simulink library "cdmalibv1p1"  (Simulink 5.0)
undefined symbols (not defined in the file or in its folder): M, N
libraries: cdmalibv1p1 x28, dspsigops x13, dspbuff3 x8, simulink3 x4, commutil2 x3, commsequence2 x1
settings Model: CovMetricSettings=d  Creator=pc  LastModifiedBy=jli

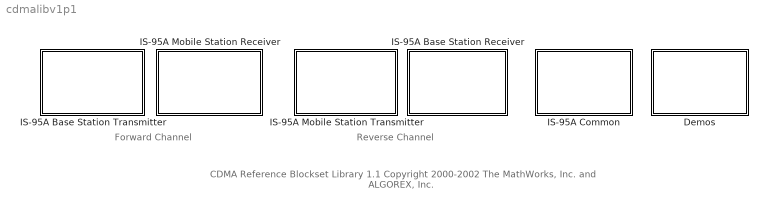
== system cdmalibv1p1 ==
  note: CDMA Reference Blockset Library 1.1
      | Copyright 2000-2002 The MathWorks, Inc. and ALGOREX, Inc.
  note: Forward Channel
  note: Reverse Channel
  Demos : Subsystem
      settings: OpenFcn=demo blocksets CDMA
      mask Type: DSP Demos
      mask Display: disp('Demos')
  IS-95A Base Station Receiver : Subsystem
      mask Display: disp('IS-95A \nBase Station\nReceiver')
  IS-95A Base Station Transmitter : Subsystem
      mask Display: disp('IS-95A \nBase Station\nTransmitter')
  IS-95A Common : Subsystem
      mask Display: disp('IS-95A \nCommon')
  IS-95A Mobile Station Receiver : Subsystem
      mask Display: disp('IS-95A \nMobile Station\nReceiver')
  IS-95A Mobile Station Transmitter : Subsystem
      mask Display: disp('IS-95A \nMobile Station\nTransmitter')

== system cdmalibv1p1/Demos ==

== system cdmalibv1p1/IS-95A Base Station Receiver ==
  IS-95A Rev Ch Viterbi Decoder : S-Function  FunctionName=sis95rcdec  Parameters=rateSet chType traceBackLenRatio decodeLenRatio  mask(IS-95A Rev Ch Viterbi Decoder){rateSet=Rate Set I, chType=Traffic, traceBackLenRatio=1, decodeLenRatio=1}
      mask prompts: rateSet "Rate set:"; chType "Channel type:"; traceBackLenRatio "Ratio of trace-back length to frame length:"; decodeLenRatio "Ratio of decoding length to frame length:"
      mask help: Perform optimum decoding for a convolutionally encoded reverse Access or Traffic channel frame.
      mask Help: web(cdmaweb);
      mask StyleString: popup(Rate Set I|Rate Set II),popup(Access|Traffic),edit,edit
      mask Display:
      | port_label('input', 1, 'Rate');
      | port_label('input', 2, 'Frame In');
      | port_label('output', 2, 'Metric');
      | port_label('output', 1, 'Frame Out');
  IS-95A Rev Ch Walsh Correlator : S-Function  FunctionName=sis95rcwalshcor  Parameters=wlshOrd numSymb  mask(IS-95A Rev Ch Walsh Correlator){wlshOrd=6, numSymb=1}
      mask prompts: wlshOrd "Walsh order:"; numSymb "Number of input symbols:"
      mask help:
      | Correlate the input sequence with a bank of Walsh sequences for the reverse Access or Traffic channel frame. The length of the input vector is
      | (Number of input symbols) * (2^Walsh order).
      mask Help: web(cdmaweb);
      mask Display: disp('IS-95A Rev Ch \nWalsh Correlator');
  IS-95A Rev Ch Walsh Demodulator : S-Function  FunctionName=sis95rcwalshdemod  Parameters=wlshOrd numSymb  mask(IS-95A Rev Ch Walsh Demodulator){wlshOrd=6, numSymb=1}
      mask prompts: wlshOrd "Walsh order:"; numSymb "Number of input symbols:"
      mask help: Perform Walsh demodulation of the received signal. The length of the input vector is (Number of input symbols) * (2^Walsh order).
      mask Help: web(cdmaweb);
      mask Display:
      | port_label('output', 1, 'Hard Dec');
      | port_label('output', 2, 'Soft Dec');
  IS-95A Rev Ch  Rake Finger : Subsystem  TreatAsAtomicUnit=on  mask(IS-95A Rev Ch Rake Finger){wlshOrd=6, outSize=1, buffSize=3, ovrSmp=8}
      mask prompts: wlshOrd "Walsh order:"; outSize "Output size (in number of walsh functions):"; buffSize "Tracking buffer size (in number of symbols):"; ovrSmp "Oversampling rate:"
      mask help: Despread the received signal with the short PN and long codes and then correlate the despread signal with all of the Walsh code sequences.
      mask Help: web(cdmaweb);
  IS-95A Rev Ch Detector : Subsystem  mask(IS-95A Rev Ch Detector){chType=Traffic, wlshOrd=6, lngcd_mask=2^41, overSamplRate=8, sampTime=1/(50*384)}
      mask prompts: chType "Channel type:"; wlshOrd "Walsh order:"; lngcd_mask "Long code mask:"; overSamplRate "Oversampling rate:"; sampTime "Sample time:"
      mask help: Perform noncoherent detection of the reverse Access or Traffic channel frame.
      mask init:
      | is95noncohdetector;
      mask Help: web(cdmaweb);
      mask StyleString: popup(Access|Traffic),edit,edit,edit,edit
  IS-95A Rev Ch Short Code Despreader : S-Function  FunctionName=sis95rcdespread  Parameters=numSymb buffSize integLen ovrSmp  mask(IS-95A Rev Ch Short Code Despreader){numSymb=1, integLen=64, buffSize=3, ovrSmp=8}
      mask prompts: numSymb "Input frame size (in number of symbols):"; integLen "Walsh size:"; buffSize "Tracking buffer size (in number of symbols):"; ovrSmp "Oversampling rate:"
      mask help: Perform despreading of the input I and Q frames with the I and Q short PN codes.
      mask Help: web(cdmaweb);
      mask Display:
      | port_label('input', 1, 'Rx I');
      | port_label('input', 2, 'Rx Q');
      | port_label('input', 3, 'PN I');
      | port_label('input', 4, 'PN Q');
      | port_label('input', 5, 'Path Delay');
      | port_label('output', 1, 'Data I');
      | port_label('output', 2, 'Data Q');

== system cdmalibv1p1/IS-95A Base Station Transmitter ==
  IS-95A Fwd Ch Convolutional Encoder : S-Function  FunctionName=sis95enc  Parameters=ch_type rate_set enc_state  mask(IS-95A Fwd Ch Convolutional Encoder){rate_set=Rate Set I, ch_type=Traffic, enc_state=[]}
      mask prompts: rate_set "Rate set:"; ch_type "Channel type:"; enc_state "Initial encoder state:"
      mask help: Convolutionally encode the bits of the forward Sync, Paging or Traffic channel frame.
      mask Help: web(cdmaweb);
      mask StyleString: popup(Rate Set I|Rate Set II),popup(Sync|Paging|Traffic),edit
      mask Display:
      | port_label('input', 1, 'Rate');
      | port_label('input', 2, 'Frame In');
  IS-95A Fwd Ch Interleaver/Deinterleaver : S-Function  FunctionName=sis95int  Parameters=ch_type intlv_tbl int_option  mask(IS-95A Fwd Ch Interleaver/Deinterleaver){ch_type=Traffic, int_select=Interleaver}
      mask prompts: ch_type "Channel type:"; int_select "Function:"
      mask help: Interleave or deinterleave the symbols of the forward Sync, Paging or Traffic Channel frame.
      mask init:
      | is95fwdchinterleaver;
      mask Help: web(cdmaweb);
      mask StyleString: popup(Sync|Paging|Traffic),popup(Interleaver|Deinterleaver)
      mask Display: disp('IS-95A Fwd Ch \nInterleaver/\nDeinterleaver');
  IS-95A Fwd Ch Repeater/Derepeater : S-Function  FunctionName=sis95rep  Parameters=ch_type rate_set rep_option  mask(IS-95A Fwd Ch Repeater/Derepeater){rate_set=Rate Set I, ch_type=Traffic, rep_select=Derepeater}
      mask prompts: rate_set "Rate set:"; ch_type "Channel type:"; rep_select "Function:"
      mask help: Repeat and puncture if necessary or derepeat the symbols of a convolutionally encoded frame for the forward Sync, Paging or Traffic channel.
      mask init:
      | is95fwdchrepeater;
      mask Help: web(cdmaweb);
      mask StyleString: popup(Rate Set I|Rate Set II),popup(Sync|Paging|Traffic),popup(Repeater|Derepeater)
      mask Display:
      | port_label('input', 1, 'Rate');
      | port_label('input', 2, 'Frame In');
  IS-95A Fwd Ch Scrambler : S-Function  FunctionName=sis95scramble  Parameters="chType  rate_set"  mask(IS-95A Fwd Ch Scrambler){rate_set=Rate Set I, chType=Traffic}
      mask prompts: rate_set "Rate set:"; chType "Channel type:"
      mask help: Scramble the symbols of the forward Paging or Traffic channel frame by the decimated long code and insert power control bits into the Traffic channel frame.
      mask Help: web(cdmaweb);
      mask StyleString: popup(Rate Set I|Rate Set II),popup(Sync|Paging|Traffic)
      mask Display:
      | port_label('input', 1, 'Rate');
      | port_label('input', 2, 'Data In');
      | port_label('input', 3, 'Long Code');
      | port_label('input', 4, 'Power Bits');
  IS-95A Fwd Ch Base Station Transmitter Interface : Subsystem  mask(IS-95A Fwd Ch Base Station Transmitter Interface){paging_rate=Full, wlshOrd=6, wlsh_indices=[0 32 2 38 23], sampTime=1/(50*384)}
      mask prompts: paging_rate "Paging channel rate:"; wlshOrd "Walsh order:"; wlsh_indices "Pilot, sync, paging, traffic and OCNS Walsh indices:"; sampTime "Sample time:"
      mask help: Combine Pilot, Sync, Paging, Traffic and Orthogonal Channel Noise Simulator (OCNS) symbols using different Walsh Code sequences.
      mask Help: web(cdmaweb);
      mask StyleString: popup(Full|Half),edit,edit,edit

== system cdmalibv1p1/IS-95A Common ==
  IS-95A CRC Generator : S-Function  FunctionName=sis95crcgen  Parameters=ch_type rate_set 1  mask(IS-95A CRC Generator){rate_set=Rate Set I, ch_type=Traffic}
      mask prompts: rate_set "Rate set:"; ch_type "Channel type:"
      mask help: Generate Cyclic Redundancy Check (CRC) bits and add them along with the tail bits to the forward or reverse Traffic channel frame.
      mask Help: web(cdmaweb);
      mask StyleString: popup(Rate Set I|Rate Set II),popup(Sync|Paging|Access|Traffic)
      mask Display:
      | port_label('input', 1, 'Rate');
      | port_label('input', 2, 'Frame In');
  IS-95A Frame Quality  Detector : Subsystem  mask(IS-95A Frame Quality Detector){rateSet=Rate Set I, chType=Traffic, rate2_metric=0.9*1.5, rate3_metric=0.85*1.5}
      mask prompts: rateSet "Rate set:"; chType "Channel type:"; rate2_metric "Metric threshold for quarter rate:"; rate3_metric "Metric threshold for eighth rate:"
      mask help: Determine the quality of a received frame of data and output the decoded data and a frame quality indicator.
      mask init:
      | is95framequalitydet;
      mask Help: web(cdmaweb);
      mask StyleString: popup(Rate Set I|Rate Set II),popup(Sync|Paging|Access|Traffic),edit,edit
  IS-95A Long Code Generator : S-Function  FunctionName=sis95lcgen2  Parameters="tx_sample_time tx_lc_init_state tx_lc_init_mask tx_lc_dec_ratio  num_symb"  mask(IS-95A Long Code Generator){num_symb=4, tx_lc_dec_ratio=1, tx_lc_init_mask=2^41, tx_lc_init_state=2^41, tx_sample_time=1/(50*384)}
      mask prompts: num_symb "Output frame size:"; tx_lc_dec_ratio "Decimation ratio:"; tx_lc_init_mask "Long code mask:"; tx_lc_init_state "Initial state:"; tx_sample_time "Sample time:"
      mask help: Generate the long code sequence used for reverse channel spreading and scrambling and forward channel scrambling.
      mask init:
      | is95longcodegenerator;
      mask Help: web(cdmaweb);
      mask Display: disp('IS-95A Long \nCode Generator');
  IS-95A Short Code Generator : S-Function  FunctionName=sis95scgen2  Parameters=numOut sampTime  mask(IS-95A Short Code Generator){numOut=64, sampTime=1/(50*384)}
      mask prompts: numOut "Output frame size:"; sampTime "Sample time:"
      mask help: Generate the I and Q short PN code sequences that are used to perform quadrature spreading of the forward or reverse channel frame. The input is a mask that determines the output of the I and Q short PN codes.
      mask Help: web(cdmaweb);
      mask Display:
      | port_label('output', 1, 'PN I');
      | port_label('output', 2, 'PN Q');
  IS-95A Syndrome Detector : S-Function  FunctionName=sis95crcgen  Parameters=chType rate_set 0  mask(IS-95A Syndrome Detector){rate_set=Rate Set I, chType=Traffic}
      mask prompts: rate_set "Rate set:"; chType "Channel type:"
      mask help: Check the CRC bits to determine the frame quality and output the decoded data and frame quality decision for all forward or reverse channels.
      mask Help: web(cdmaweb);
      mask StyleString: popup(Rate Set I|Rate Set II),popup(Sync|Paging|Access|Traffic)
      mask Display:
      | port_label('input', 1, 'Rate');
      | port_label('input', 2, 'Frame In');
      | port_label('output', 1, 'Frame Out');
      | port_label('output', 2, 'Frame Error');
  IS-95A Walsh Code Generator : S-Function  FunctionName=sis95wcgen2  Parameters=wlshOrd wlshIndices st  mask(IS-95A Walsh Code Generator){wlshOrd=6, wlshIndices=[0 32 2 38 23], st=1/(50*384)}
      mask prompts: wlshOrd "Walsh order:"; wlshIndices "Walsh indices:"; st "Sample time:"
      mask help: Generate the Walsh code sequences corresponding to the specified Walsh order and indices.
      mask Help: web(cdmaweb);
      mask Display: disp('IS-95A Walsh \nCode Generator');

== system cdmalibv1p1/IS-95A Mobile Station Receiver ==
  IS-95A Fwd Ch Descrambler : Subsystem  mask(IS-95A Fwd Ch Descrambler){rateSet=Rate Set I, rake_buff_size=3}
      mask prompts: rateSet "Rate set:"; rake_buff_size "Tracking buffer size:"
      mask help: Perform power bit extraction and descrambling for each rake finger and combine the signals from all the fingers.
      mask init:
      | is95fwdchdescramble;
      mask Help: web(cdmaweb);
      mask StyleString: popup(Rate Set I|Rate Set II),edit
  IS-95A Fwd Ch Power Bit Extractor : Subsystem  TreatAsAtomicUnit=on  mask(IS-95A Fwd Ch Power Bit Extractor){rateSet=Rate Set I, num_symb=1, init_loc=0}
      mask prompts: rateSet "Rate set:"; num_symb "Input frame size:"; init_loc "Initial power bit location:"
      mask help: Extract power control bits from the forward Traffic channel frame.
      mask init:
      | is95fwdchpwrbitext;
      mask Help: web(cdmaweb);
      mask StyleString: popup(Rate Set I|Rate Set II),edit,edit
  IS-95A Fwd Ch Rake Demodulator : S-Function  FunctionName=sis95rakedemod  Parameters=num_symb 4  mask(IS-95A Fwd Ch Rake Demodulator){num_symb=1}
      mask prompts: num_symb "Input frame size per finger:"
      mask help: Demodulate the data obtained from the four rake receiver fingers utilizing the pilot signal for each finger.
      mask Help: web(cdmaweb);
      mask Display:
      | port_label('input', 1, 'Pilot I');
      | port_label('input', 2, 'Pilot Q');
      | port_label('input', 3, 'Data I');
      | port_label('input', 4, 'Data Q');
      | port_label('output', 1, 'Finger 1');
      | port_label('output', 2, 'Finger 2');
      | port_label('output', 3, 'Finger 3');
      | port_label('output', 4, 'Finger 4');
  IS-95A Fwd Ch Viterbi Decoder : S-Function  FunctionName=sis95dec  Parameters=rateSet chType traceBackLenRatio decodeLenRatio  mask(IS-95A Fwd Ch Viterbi Decoder){rateSet=Rate Set I, chType=Traffic, traceBackLenRatio=1, decodeLenRatio=1}
      mask prompts: rateSet "Rate set:"; chType "Channel type:"; traceBackLenRatio "Ratio of trace-back length to frame length:"; decodeLenRatio "Ratio of decoding length to frame length:"
      mask help: Perform optimum decoding for a convolutionally encoded forward Sync, Paging or Traffic channel frame.
      mask Help: web(cdmaweb);
      mask StyleString: popup(Rate Set I|Rate Set II),popup(Sync|Paging|Traffic),edit,edit
      mask Display:
      | port_label('input', 1, 'Rate');
      | port_label('input', 2, 'Frame In');
      | port_label('output', 2, 'Metric');
      | port_label('output', 1, 'Frame Out');
  IS-95A Fwd Ch  Rake Finger : Subsystem  TreatAsAtomicUnit=on  mask(IS-95A Fwd Ch Rake Finger){wlshOrd=6, numSymb=1, buffSize=3, ovrSmp=8}
      mask prompts: wlshOrd "Walsh order:"; numSymb "Input frame size (in number of symbols):"; buffSize "Tracking buffer size (in number of symbols):"; ovrSmp "Oversampling rate:"
      mask help: Correlate the input signal over each Walsh code interval with the short PN code and the Walsh code sequences supplied.
      mask init:
      | is95fwdchrakefinger;
      mask Help: web(cdmaweb);
  IS-95A Fwd Ch Detector : Subsystem  mask(IS-95A Fwd Ch Detector){rateSet=Rate Set I, numSymb=1, wlshOrd=6, rake_buff_size=3, rake_oversamp=8, sampTime=1/(50*384)}
      mask prompts: rateSet "Rate set:"; numSymb "Input frame size (in number of symbols):"; wlshOrd "Walsh order:"; rake_buff_size "Tracking buffer size (in number of symbols):"; rake_oversamp "Oversampling rate:"; sampTime "Sample time:"
      mask help: Perform despreading, demodulation and rake combining of the received signal.
      mask init:
      | is95cohdetector;
      mask Help: web(cdmaweb);
      mask StyleString: popup(Rate Set I|Rate Set II),edit,edit,edit,edit,edit

== system cdmalibv1p1/IS-95A Mobile Station Transmitter ==
  IS-95A Rev Ch Burst Randomizer : S-Function  FunctionName=sis95rcrandomizer  Parameters=chType initLCSt  mask(IS-95A Rev Ch Burst Randomizer){chType=Traffic, initLCSt=[]}
      mask prompts: chType "Channel type:"; initLCSt "Randomizer initial state:"
      mask help: Generate a pseudorandom masking pattern of 0's and 1's that can be used to mask redundant power groups.
      mask Help: web(cdmaweb);
      mask StyleString: popup(Access|Traffic),edit
      mask Display:
      | port_label('input', 1, 'Rate');
      | port_label('input', 2, 'Long Code');
  IS-95A Rev Ch Convolutional Encoder : S-Function  FunctionName=sis95rcenc  Parameters=ch_type rate_set enc_state  mask(IS-95A Rev Ch Convolutional Encoder){rate_set=Rate Set I, ch_type=Traffic, enc_state=[]}
      mask prompts: rate_set "Rate set:"; ch_type "Channel type:"; enc_state "Initial encoder state:"
      mask help: Convolutionally encode the bits of the reverse Access or Traffic channel frame.
      mask Help: web(cdmaweb);
      mask StyleString: popup(Rate Set I|Rate Set II),popup(Access|Traffic),edit
      mask Display:
      | port_label('input', 1, 'Rate');
      | port_label('input', 2, 'Frame In');
  IS-95A Rev Ch Interleaver/Deinterleaver : S-Function  FunctionName=sis95rcint  Parameters=ch_type rlinttable int_option  mask(IS-95A Rev Ch Interleaver/Deinterleaver){ch_type=Traffic, int_select=Interleaver}
      mask prompts: ch_type "Channel type:"; int_select "Function:"
      mask help: Interleave or deinterleave the symbols of the reverse Access or Traffic channel frame.
      mask init:
      | is95revchinterleaver;
      mask Help: web(cdmaweb);
      mask StyleString: popup(Access|Traffic),popup(Interleaver|Deinterleaver)
      mask Display:
      | port_label('input', 1, 'Rate');
      | port_label('input', 2, 'Frame In');
  IS-95A Rev Ch Repeater/Derepeater : S-Function  FunctionName=sis95rcrep  Parameters=ch_type rep_option  mask(IS-95A Rev Ch Repeater/Derepeater){ch_type=Traffic, rep_select=Derepeater}
      mask prompts: ch_type "Channel type:"; rep_select "Function:"
      mask help: Repeat or derepeat the symbols of the convolutionally encoded frame for the reverse Access or Traffic channel.
      mask init:
      | is95revchrepeater;
      mask Help: web(cdmaweb);
      mask StyleString: popup(Access|Traffic),popup(Repeater|Derepeater)
      mask Display:
      | port_label('input', 1, 'Rate');
      | port_label('input', 2, 'Frame In');
  IS-95A Rev Ch Walsh Modulator : S-Function  FunctionName=sis95walshmod  Parameters=walshOrder numSymb  mask(IS-95A Rev Ch Walsh Modulator){walshOrder=6, numSymb=6}
      mask prompts: walshOrder "Walsh order:"; numSymb "Input vector length:"
      mask help:
      | Modulate the input data symbols with the Walsh code sequences.
      | The length of the input vector must be an integer multiple of the Walsh order.
      mask Help: web(cdmaweb);
      mask Display: disp('IS-95A Rev Ch \nWalsh Modulator');
  IS-95A Rev Ch Walsh Modulation and Spreading : Subsystem  mask(IS-95A Rev Ch Walsh Modulation and Spreading){chType=Traffic, lngCdMask=1, wlshOrd=6, sampTime=1/(50*384)}
      mask prompts: chType "Channel type:"; lngCdMask "Long code mask:"; wlshOrd "Walsh order:"; sampTime "Sample time:"
      mask help: Perform Walsh code modulation, spreading with the long code, and power group randomization on a reverse Access or Traffic channel frame.
      mask init:
      | is95revchmodspread;
      mask Help: web(cdmaweb);
      mask StyleString: popup(Access|Traffic),edit,edit,edit

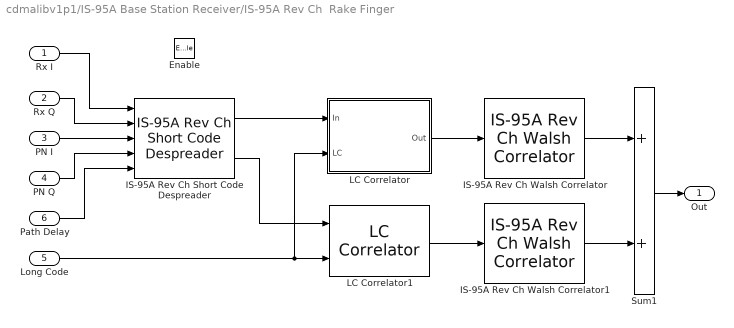
== system cdmalibv1p1/IS-95A Base Station Receiver/IS-95A Rev Ch  Rake Finger ==
  Rx I : Inport
  Rx Q : Inport  Port=2
  PN I : Inport  Port=3
  PN Q : Inport  Port=4
  Long Code : Inport  Port=5
  Path Delay : Inport  Port=6
  Enable : EnablePort
  IS-95A Rev Ch Walsh Correlator : cdmalibv1p1/IS-95A Base Station Receiver/IS-95A Rev Ch Walsh Correlator  wlshOrd=wlshOrd  numSymb=outSize
  IS-95A Rev Ch Walsh Correlator1 : cdmalibv1p1/IS-95A Base Station Receiver/IS-95A Rev Ch Walsh Correlator  wlshOrd=wlshOrd  numSymb=outSize
  IS-95A Rev Ch Short Code Despreader : cdmalibv1p1/IS-95A Base Station Receiver/IS-95A Rev Ch Short Code Despreader  numSymb=outSize  integLen=2^wlshOrd  buffSize=buffSize  ovrSmp=ovrSmp
  LC Correlator : Subsystem
  LC Correlator1 : cdmalibv1p1/IS-95A Base Station Receiver/IS-95A Rev Ch  Rake Finger/LC Correlator
      settings: RTWFcnNameOpts=Auto  RTWFileNameOpts=Auto
  Sum1 : Sum  SaturateOnIntegerOverflow=on  InputSameDT=on
  Out : Outport  InitialOutput=0
  wires:
  Long Code/1 -> LC Correlator/2(LC), LC Correlator1/2
  IS-95A Rev Ch Short Code Despreader/1 -> LC Correlator/1(In)
  Path Delay/1 -> IS-95A Rev Ch Short Code Despreader/5
  PN Q/1 -> IS-95A Rev Ch Short Code Despreader/4
  PN I/1 -> IS-95A Rev Ch Short Code Despreader/3
  Rx Q/1 -> IS-95A Rev Ch Short Code Despreader/2
  Rx I/1 -> IS-95A Rev Ch Short Code Despreader/1
  IS-95A Rev Ch Short Code Despreader/2 -> LC Correlator1/1
  IS-95A Rev Ch Walsh Correlator/1 -> Sum1/1
  Sum1/1 -> Out/1
  IS-95A Rev Ch Walsh Correlator1/1 -> Sum1/2
  LC Correlator1/1 -> IS-95A Rev Ch Walsh Correlator1/1
  LC Correlator/1(Out) -> IS-95A Rev Ch Walsh Correlator/1

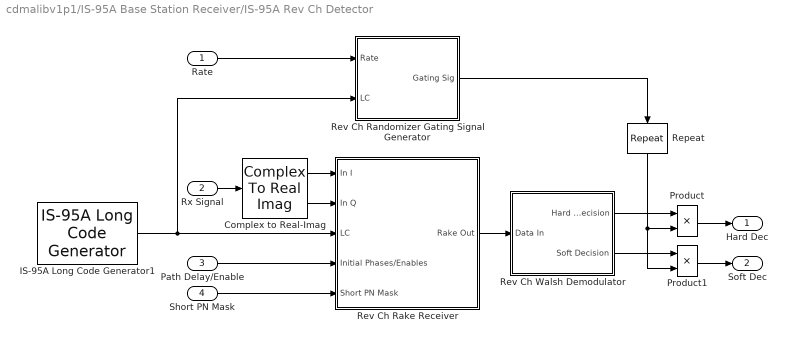
== system cdmalibv1p1/IS-95A Base Station Receiver/IS-95A Rev Ch Detector ==
  Rate : Inport
  Rx Signal : Inport  Port=2
  Path Delay/Enable : Inport  Port=3
  Short PN Mask : Inport  Port=4
  Complex to Real-Imag : ComplexToRealImag
  IS-95A Long Code Generator1 : cdmalibv1p1/IS-95A Common/IS-95A Long Code Generator  num_symb=N*(2^wlshOrd)*4  tx_lc_dec_ratio=1  tx_lc_init_mask=lngcd_mask  tx_lc_init_state=[]  tx_sample_time=N*4*sampTime
  Product : Product  SaturateOnIntegerOverflow=on  InputSameDT=on
  Product1 : Product  SaturateOnIntegerOverflow=on  InputSameDT=on
  Repeat : dspsigops/Repeat  Orientation=down  N=36  ic=0  mode=Maintain input frame rate
  Rev Ch Rake Receiver : Subsystem
  Rev Ch Randomizer Gating Signal Generator : Subsystem
  Rev Ch Walsh Demodulator : Subsystem  mask(IS95A NonCoh Walsh Demod){inSize=N, off=(M+1)*N, wlshOrder=wlshOrd}
      mask prompts: inSize "Input Size (in No of Walsh Functions)"; off "Input Delay (in No of Walsh Functions)"; wlshOrder "Walsh Order"
      mask help: Performs Walsh demodulation of the signal after combining the output of the rake fingers.
      mask Help: web(cdmaweb);
  Hard Dec : Outport  InitialOutput=0
  Soft Dec : Outport  Port=2  InitialOutput=0
  wires:
  IS-95A Long Code Generator1/1 -> Rev Ch Rake Receiver/3(LC), Rev Ch Randomizer Gating Signal Generator/2(LC)
  Complex to Real-Imag/1 -> Rev Ch Rake Receiver/1(In I)
  Rev Ch Randomizer Gating Signal Generator/1(Gating Sig) -> Repeat/1
  Complex to Real-Imag/2 -> Rev Ch Rake Receiver/2(In Q)
  Path Delay/Enable/1 -> Rev Ch Rake Receiver/4(Initial Phases/Enables)
  Rev Ch Rake Receiver/1(Rake Out) -> Rev Ch Walsh Demodulator/1(Data In)
  Short PN Mask/1 -> Rev Ch Rake Receiver/5(Short PN Mask)
  Rx Signal/1 -> Complex to Real-Imag/1
  Repeat/1 -> Product/2, Product1/2
  Rev Ch Walsh Demodulator/2(Soft Decision) -> Product1/1
  Rev Ch Walsh Demodulator/1(Hard Decision) -> Product/1
  Product/1 -> Hard Dec/1
  Product1/1 -> Soft Dec/1
  Rate/1 -> Rev Ch Randomizer Gating Signal Generator/1(Rate)

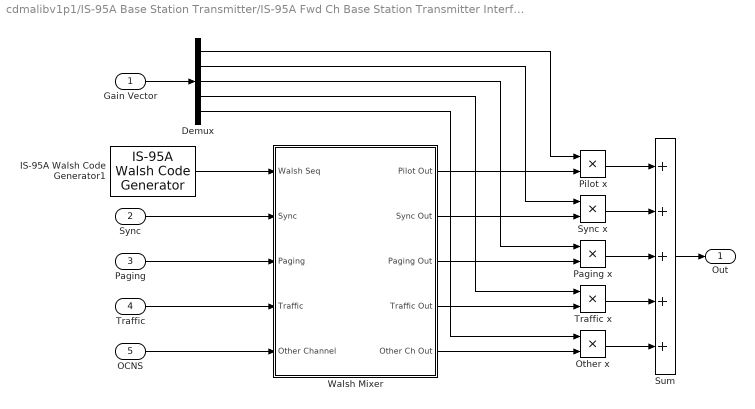
== system cdmalibv1p1/IS-95A Base Station Transmitter/IS-95A Fwd Ch Base Station Transmitter Interface ==
  Gain Vector : Inport
  Sync : Inport  Port=2
  Paging : Inport  Port=3
  Traffic : Inport  Port=4
  OCNS : Inport  Port=5
  Demux : Demux  Outputs=5
  IS-95A Walsh Code Generator1 : cdmalibv1p1/IS-95A Common/IS-95A Walsh Code Generator  wlshOrd=wlshOrd  wlshIndices=wlsh_indices  st=sampTime
  Other x : Product  Inputs=**  SaturateOnIntegerOverflow=on  InputSameDT=on
  Paging x : Product  Inputs=**  SaturateOnIntegerOverflow=on  InputSameDT=on
  Pilot x : Product  Inputs=**  SaturateOnIntegerOverflow=on  InputSameDT=on
  Sum : Sum  Inputs=+++++  SaturateOnIntegerOverflow=on  InputSameDT=on
  Sync x : Product  Inputs=**  SaturateOnIntegerOverflow=on  InputSameDT=on
  Traffic x : Product  Inputs=**  SaturateOnIntegerOverflow=on  InputSameDT=on
  Walsh Mixer : Subsystem
  Out : Outport  InitialOutput=0
  wires:
  IS-95A Walsh Code Generator1/1 -> Walsh Mixer/1(Walsh Seq)
  Walsh Mixer/5(Other Ch Out) -> Other x/2
  Walsh Mixer/4(Traffic Out) -> Traffic x/2
  Walsh Mixer/3(Paging Out) -> Paging x/2
  Walsh Mixer/2(Sync Out) -> Sync x/2
  Walsh Mixer/1(Pilot Out) -> Pilot x/2
  OCNS/1 -> Walsh Mixer/5(Other Channel)
  Traffic/1 -> Walsh Mixer/4(Traffic)
  Paging/1 -> Walsh Mixer/3(Paging)
  Sync/1 -> Walsh Mixer/2(Sync)
  Other x/1 -> Sum/5
  Traffic x/1 -> Sum/4
  Paging x/1 -> Sum/3
  Sync x/1 -> Sum/2
  Pilot x/1 -> Sum/1
  Sum/1 -> Out/1
  Gain Vector/1 -> Demux/1
  Demux/5 -> Other x/1
  Demux/4 -> Traffic x/1
  Demux/3 -> Paging x/1
  Demux/2 -> Sync x/1
  Demux/1 -> Pilot x/1

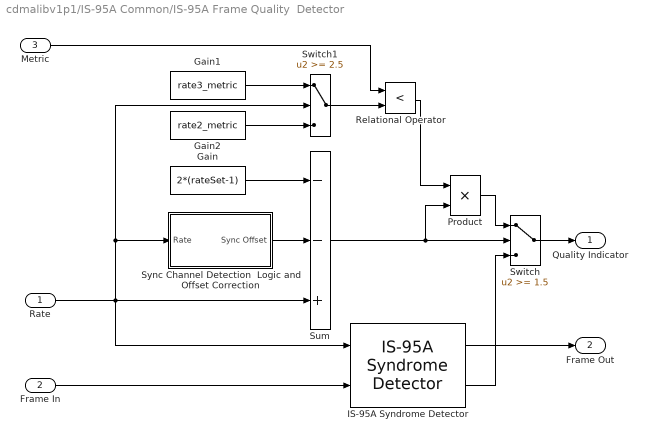
== system cdmalibv1p1/IS-95A Common/IS-95A Frame Quality  Detector ==
  Rate : Inport
  Frame In : Inport  Port=2
  Metric : Inport  Port=3
  Gain : Constant  Value=2*(rateSet-1)
  Gain1 : Constant  Value=rate3_metric
  Gain2 : Constant  Value=rate2_metric
  IS-95A Syndrome Detector : cdmalibv1p1/IS-95A Common/IS-95A Syndrome Detector  rate_set=Rate Set I  chType=Traffic
  Product : Product  SaturateOnIntegerOverflow=on  InputSameDT=on
  Relational Operator : RelationalOperator  Operator=<
  Sum : Sum  Inputs=--+  SaturateOnIntegerOverflow=on  InputSameDT=on
  Switch : Switch  Threshold=1.5
  Switch1 : Switch  Threshold=2.5
  Sync Channel Detection  Logic and Offset Correction : Subsystem
  Quality Indicator : Outport  InitialOutput=0
  Frame Out : Outport  Port=2  InitialOutput=0
  wires:
  Sync Channel Detection  Logic and Offset Correction/1(Sync Offset) -> Sum/2
  Rate/1 -> IS-95A Syndrome Detector/1, Sum/3, Sync Channel Detection  Logic and Offset Correction/1(Rate), Switch1/2
  Frame In/1 -> IS-95A Syndrome Detector/2
  IS-95A Syndrome Detector/1 -> Frame Out/1
  Gain/1 -> Sum/1
  Switch1/1 -> Relational Operator/2
  Metric/1 -> Relational Operator/1
  Gain2/1 -> Switch1/3
  Gain1/1 -> Switch1/1
  IS-95A Syndrome Detector/2 -> Switch/3
  Sum/1 -> Switch/2, Product/2
  Product/1 -> Switch/1
  Switch/1 -> Quality Indicator/1
  Relational Operator/1 -> Product/1

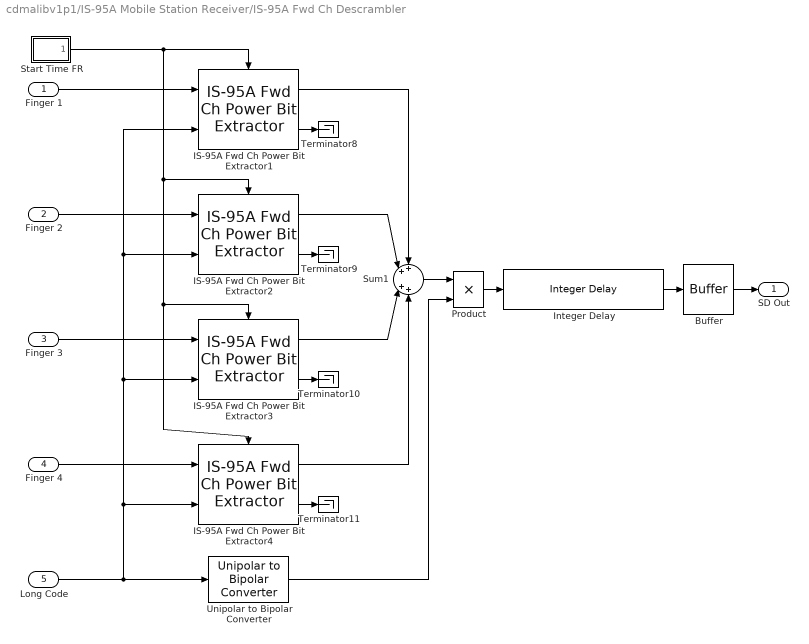
== system cdmalibv1p1/IS-95A Mobile Station Receiver/IS-95A Fwd Ch Descrambler ==
  Finger 1 : Inport
  Finger 2 : Inport  Port=2
  Finger 3 : Inport  Port=3
  Finger 4 : Inport  Port=4
  Long Code : Inport  Port=5
  Buffer : dspbuff3/Buffer  N=384  V=0  ic=0
  IS-95A Fwd Ch Power Bit Extractor{1..4} (4 alike) : cdmalibv1p1/IS-95A Mobile Station Receiver/IS-95A Fwd Ch Power Bit Extractor  rateSet=Rate Set I  num_symb=1  init_loc=0
  Integer Delay : dspsigops/Integer Delay  delay=384 - rake_buff_size  ic=0
  Product : Product  SaturateOnIntegerOverflow=on  InputSameDT=on
  Start Time FR : Subsystem
  Sum1 : Sum  Inputs=++|++  SaturateOnIntegerOverflow=on  InputSameDT=on
  Terminator{8..11} (4 alike) : Terminator
  Unipolar to Bipolar Converter : commutil2/Unipolar to Bipolar Converter  M=2  polarity=Negative
  SD Out : Outport  InitialOutput=0
  wires:
  IS-95A Fwd Ch Power Bit Extractor3/1 -> Sum1/3
  IS-95A Fwd Ch Power Bit Extractor2/1 -> Sum1/2
  IS-95A Fwd Ch Power Bit Extractor1/1 -> Sum1/1
  IS-95A Fwd Ch Power Bit Extractor4/1 -> Sum1/4
  Long Code/1 -> IS-95A Fwd Ch Power Bit Extractor1/2, IS-95A Fwd Ch Power Bit Extractor2/2, IS-95A Fwd Ch Power Bit Extractor3/2, IS-95A Fwd Ch Power Bit Extractor4/2, Unipolar to Bipolar Converter/1
  Unipolar to Bipolar Converter/1 -> Product/2
  Integer Delay/1 -> Buffer/1
  Buffer/1 -> SD Out/1
  Product/1 -> Integer Delay/1
  IS-95A Fwd Ch Power Bit Extractor4/2 -> Terminator11/1
  Finger 4/1 -> IS-95A Fwd Ch Power Bit Extractor4/1
  IS-95A Fwd Ch Power Bit Extractor3/2 -> Terminator10/1
  Finger 3/1 -> IS-95A Fwd Ch Power Bit Extractor3/1
  IS-95A Fwd Ch Power Bit Extractor2/2 -> Terminator9/1
  Finger 2/1 -> IS-95A Fwd Ch Power Bit Extractor2/1
  Sum1/1 -> Product/1
  IS-95A Fwd Ch Power Bit Extractor1/2 -> Terminator8/1
  Finger 1/1 -> IS-95A Fwd Ch Power Bit Extractor1/1
  Start Time FR/1(Enable) -> IS-95A Fwd Ch Power Bit Extractor4/Enable, IS-95A Fwd Ch Power Bit Extractor3/Enable, IS-95A Fwd Ch Power Bit Extractor2/Enable, IS-95A Fwd Ch Power Bit Extractor1/Enable

== system cdmalibv1p1/IS-95A Mobile Station Receiver/IS-95A Fwd Ch Power Bit Extractor ==
  Finger In : Inport
  Long Code : Inport  Port=2
  Enable : EnablePort  StatesWhenEnabling=reset
  IS-95A Fwd Ch Power Bit Extractor : S-Function  FunctionName=sis95pwrbitext  Parameters=rateSet num_symb init_loc  mask(IS-95A Fwd Ch Power Bit Extractor){rateSet=Rate Set I, num_symb=num_symb, init_loc=init_loc}
      mask prompts: rateSet "Rate set:"; num_symb "Input frame size:"; init_loc "Initial power bit location:"
      mask help: Extracts power bits from the received data.
      mask Help: web(cdmaweb);
      mask StyleString: popup(Rate Set I|Rate Set II),edit,edit
      mask Display:
      | port_label('input', 1, 'In');
      | port_label('input', 2, 'Long Code');
      | port_label('output', 1, 'Out');
      | port_label('output', 2, 'Power Bits');
  Data Out : Outport  InitialOutput=0
  Power Bits : Outport  Port=2  InitialOutput=0
  wires:
  IS-95A Fwd Ch Power Bit Extractor/1 -> Data Out/1
  IS-95A Fwd Ch Power Bit Extractor/2 -> Power Bits/1
  Finger In/1 -> IS-95A Fwd Ch Power Bit Extractor/1
  Long Code/1 -> IS-95A Fwd Ch Power Bit Extractor/2

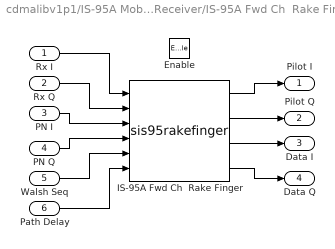
== system cdmalibv1p1/IS-95A Mobile Station Receiver/IS-95A Fwd Ch  Rake Finger ==
  Rx I : Inport
  Rx Q : Inport  Port=2
  PN I : Inport  Port=3
  PN Q : Inport  Port=4
  Walsh Seq : Inport  Port=5
  Path Delay : Inport  Port=6
  Enable : EnablePort  StatesWhenEnabling=reset
  IS-95A Fwd Ch  Rake Finger : S-Function  FunctionName=sis95rakefinger  Parameters=numSymb buffSize integLen ovrSmp  mask(IS-95A Fwd Ch Rake Finger){wlshOrd=wlshOrd, numSymb=numSymb, buffSize=buffSize, ovrSmp=ovrSmp}
      mask prompts: wlshOrd "Walsh order:"; numSymb "Input frame size (in number of symbols):"; buffSize "Tracking buffer size (in number of symbols):"; ovrSmp "Oversampling rate:"
      mask help: Correlates the input signal over each Walsh code interval with the short PN code and Walsh code sequences supplied.
      mask init:
      | integLen=2^wlshOrd;
      mask Help: web(cdmaweb);
      mask Display:
      | port_label('input', 1, 'In I');
      | port_label('input', 2, 'In Q');
      | port_label('input', 3, 'PN I');
      | port_label('input', 4, 'PN Q');
      | port_label('input', 5, 'Walsh Seq');
      | port_label('input', 6, 'Path Delay');
      | port_label('output', 1, 'Pilot I');
      | port_label('output', 2, 'Pilot Q');
      | port_label('output', 3, 'Out I');
      | port_label('output', 4, 'Out Q');
  Pilot I : Outport  InitialOutput=0
  Pilot Q : Outport  Port=2  InitialOutput=0
  Data I : Outport  Port=3  InitialOutput=0
  Data Q : Outport  Port=4  InitialOutput=0
  wires:
  PN I/1 -> IS-95A Fwd Ch  Rake Finger/3
  PN Q/1 -> IS-95A Fwd Ch  Rake Finger/4
  Walsh Seq/1 -> IS-95A Fwd Ch  Rake Finger/5
  Path Delay/1 -> IS-95A Fwd Ch  Rake Finger/6
  Rx Q/1 -> IS-95A Fwd Ch  Rake Finger/2
  Rx I/1 -> IS-95A Fwd Ch  Rake Finger/1
  IS-95A Fwd Ch  Rake Finger/2 -> Pilot Q/1
  IS-95A Fwd Ch  Rake Finger/1 -> Pilot I/1
  IS-95A Fwd Ch  Rake Finger/3 -> Data I/1
  IS-95A Fwd Ch  Rake Finger/4 -> Data Q/1

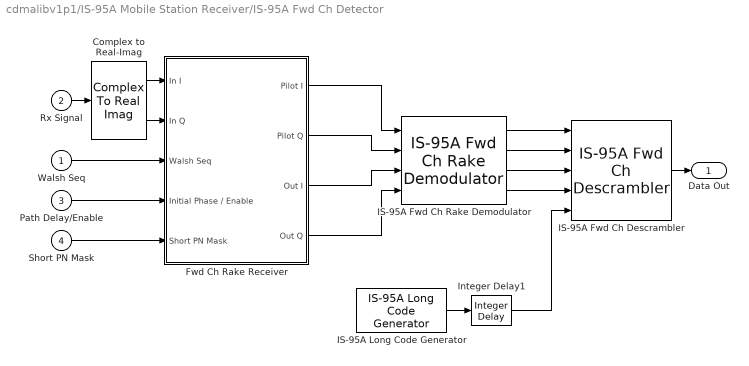
== system cdmalibv1p1/IS-95A Mobile Station Receiver/IS-95A Fwd Ch Detector ==
  Walsh Seq : Inport
  Rx Signal : Inport  Port=2
  Path Delay/Enable : Inport  Port=3
  Short PN Mask : Inport  Port=4
  Complex to Real-Imag : ComplexToRealImag
  "Fwd Ch Rake Receiver " : Subsystem
  IS-95A Fwd Ch Descrambler : cdmalibv1p1/IS-95A Mobile Station Receiver/IS-95A Fwd Ch Descrambler  rateSet=Rate Set I  rake_buff_size=rake_buff_size
  IS-95A Fwd Ch Rake Demodulator : cdmalibv1p1/IS-95A Mobile Station Receiver/IS-95A Fwd Ch Rake Demodulator  num_symb=1
  IS-95A Long Code Generator : cdmalibv1p1/IS-95A Common/IS-95A Long Code Generator  num_symb=1  tx_lc_dec_ratio=2^ wlshOrd  tx_lc_init_mask=2^41  tx_lc_init_state=2^41  tx_sample_time=sampTime
  Integer Delay1 : dspsigops/Integer Delay  delay=rake_buff_size  ic=0
  Data Out : Outport  InitialOutput=0
  wires:
  "Fwd Ch Rake Receiver "/4(Out Q) -> IS-95A Fwd Ch Rake Demodulator/4
  "Fwd Ch Rake Receiver "/3(Out I) -> IS-95A Fwd Ch Rake Demodulator/3
  "Fwd Ch Rake Receiver "/2(Pilot Q) -> IS-95A Fwd Ch Rake Demodulator/2
  "Fwd Ch Rake Receiver "/1(Pilot I) -> IS-95A Fwd Ch Rake Demodulator/1
  IS-95A Fwd Ch Descrambler/1 -> Data Out/1
  Path Delay/Enable/1 -> "Fwd Ch Rake Receiver "/4(Initial Phase / Enable)
  Walsh Seq/1 -> "Fwd Ch Rake Receiver "/3(Walsh Seq)
  Complex to Real-Imag/1 -> "Fwd Ch Rake Receiver "/1(In I)
  Complex to Real-Imag/2 -> "Fwd Ch Rake Receiver "/2(In Q)
  Short PN Mask/1 -> "Fwd Ch Rake Receiver "/5(Short PN Mask)
  Rx Signal/1 -> Complex to Real-Imag/1
  IS-95A Long Code Generator/1 -> Integer Delay1/1
  Integer Delay1/1 -> IS-95A Fwd Ch Descrambler/5
  IS-95A Fwd Ch Rake Demodulator/4 -> IS-95A Fwd Ch Descrambler/4
  IS-95A Fwd Ch Rake Demodulator/3 -> IS-95A Fwd Ch Descrambler/3
  IS-95A Fwd Ch Rake Demodulator/2 -> IS-95A Fwd Ch Descrambler/2
  IS-95A Fwd Ch Rake Demodulator/1 -> IS-95A Fwd Ch Descrambler/1

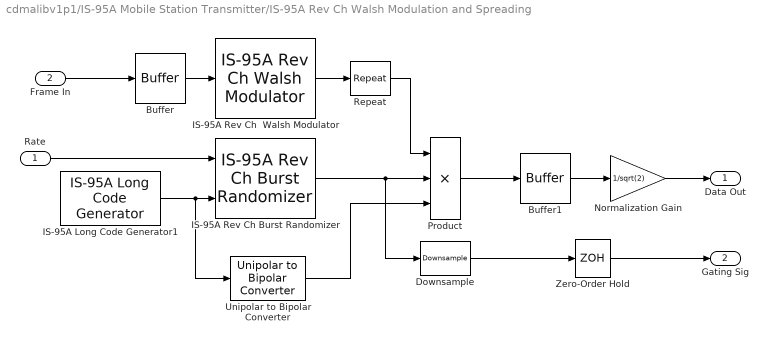
== system cdmalibv1p1/IS-95A Mobile Station Transmitter/IS-95A Rev Ch Walsh Modulation and Spreading ==
  Rate : Inport
  Frame In : Inport  Port=2
  Buffer : dspbuff3/Buffer  N=wlshOrd  V=0  ic=0
  Buffer1 : dspbuff3/Buffer  N=2^wlshOrd  V=0  ic=0
  Downsample : dspsigops/Downsample  N=(2^wlshOrd)*4  phase=0  ic=0  smode=Allow multirate  fmode=Maintain input frame rate
  IS-95A Long Code Generator1 : cdmalibv1p1/IS-95A Common/IS-95A Long Code Generator  num_symb=4*(2^wlshOrd)  tx_lc_dec_ratio=1  tx_lc_init_mask=lngCdMask  tx_lc_init_state=[]  tx_sample_time=4*sampTime
  IS-95A Rev Ch Burst Randomizer : cdmalibv1p1/IS-95A Mobile Station Transmitter/IS-95A Rev Ch Burst Randomizer  chType=Traffic  initLCSt=[]
  IS-95A Rev Ch  Walsh Modulator : cdmalibv1p1/IS-95A Mobile Station Transmitter/IS-95A Rev Ch Walsh Modulator  walshOrder=wlshOrd  numSymb=wlshOrd
  Normalization Gain : Gain  Gain=1/sqrt(2)  SaturateOnIntegerOverflow=on
  Product : Product  Inputs=3  SaturateOnIntegerOverflow=on  InputSameDT=on
  Repeat : dspsigops/Repeat  N=4  ic=0  mode=Maintain input frame rate
  Unipolar to Bipolar Converter : commutil2/Unipolar to Bipolar Converter  M=2  polarity=Negative
  Zero-Order Hold : ZeroOrderHold  SampleTime=sampTime
  Data Out : Outport  InitialOutput=0
  Gating Sig : Outport  Port=2  InitialOutput=0
  wires:
  IS-95A Long Code Generator1/1 -> IS-95A Rev Ch Burst Randomizer/2, Unipolar to Bipolar Converter/1
  IS-95A Rev Ch  Walsh Modulator/1 -> Repeat/1
  IS-95A Rev Ch Burst Randomizer/1 -> Downsample/1, Product/2
  Rate/1 -> IS-95A Rev Ch Burst Randomizer/1
  Repeat/1 -> Product/1
  Product/1 -> Buffer1/1
  Frame In/1 -> Buffer/1
  Buffer/1 -> IS-95A Rev Ch  Walsh Modulator/1
  Unipolar to Bipolar Converter/1 -> Product/3
  Normalization Gain/1 -> Data Out/1
  Buffer1/1 -> Normalization Gain/1
  Zero-Order Hold/1 -> Gating Sig/1
  Downsample/1 -> Zero-Order Hold/1

== system cdmalibv1p1/IS-95A Base Station Receiver/IS-95A Rev Ch  Rake Finger/LC Correlator ==
  In : Inport
  LC : Inport  Port=2
  Buffer : dspbuff3/Buffer  N=4*outSize*(2^wlshOrd)  V=0  ic=0
  Derepeat : commsequence2/Derepeat  N=4  ic=0  mode=Maintain input frame rate
  Product : Product  SaturateOnIntegerOverflow=on  InputSameDT=on
  Out : Outport  InitialOutput=0
  wires:
  Derepeat/1 -> Out/1
  Buffer/1 -> Product/1
  Product/1 -> Derepeat/1
  In/1 -> Buffer/1
  LC/1 -> Product/2

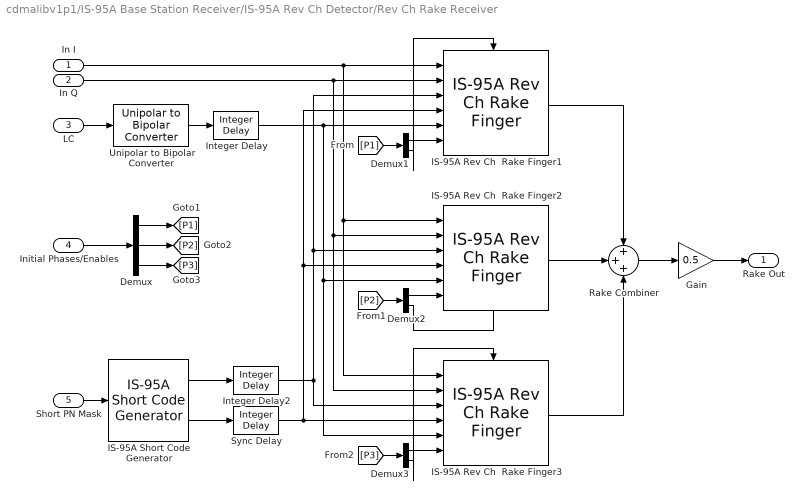
== system cdmalibv1p1/IS-95A Base Station Receiver/IS-95A Rev Ch Detector/Rev Ch Rake Receiver ==
  In I : Inport
  In Q : Inport  Port=2
  LC : Inport  Port=3
  Initial Phases/Enables : Inport  Port=4
  Short PN Mask : Inport  Port=5
  Demux : Demux  Outputs=3
  Demux1 : Demux  Outputs=2
  Demux2 : Demux  Outputs=2
  Demux3 : Demux  Outputs=2
  Gain : Gain  Gain=0.5  SaturateOnIntegerOverflow=on
  IS-95A Rev Ch  Rake Finger1 : cdmalibv1p1/IS-95A Base Station Receiver/IS-95A Rev Ch  Rake Finger  wlshOrd=wlshOrd  outSize=N  buffSize=M*4*N  ovrSmp=overSamplRate
  IS-95A Rev Ch  Rake Finger2 : cdmalibv1p1/IS-95A Base Station Receiver/IS-95A Rev Ch  Rake Finger  wlshOrd=wlshOrd  outSize=N  buffSize=M*4*N  ovrSmp=overSamplRate
  IS-95A Rev Ch  Rake Finger3 : cdmalibv1p1/IS-95A Base Station Receiver/IS-95A Rev Ch  Rake Finger  wlshOrd=wlshOrd  outSize=N  buffSize=M*4*N  ovrSmp=overSamplRate
  IS-95A Short Code Generator : cdmalibv1p1/IS-95A Common/IS-95A Short Code Generator  numOut=2^wlshOrd  sampTime=1/(50*384)
  Integer Delay : dspsigops/Integer Delay  delay=N*(2^wlshOrd)*4*(1 + M)  ic=0
  Integer Delay2 : dspsigops/Integer Delay  delay=M*4*N*(2^wlshOrd)  ic=0
  Rake Combiner : Sum  Inputs=+++  SaturateOnIntegerOverflow=on  InputSameDT=on
  Sync Delay : dspsigops/Integer Delay  delay=M*4*N*(2^wlshOrd)  ic=0
  Unipolar to Bipolar Converter : commutil2/Unipolar to Bipolar Converter  M=2  polarity=Negative
  Rake Out : Outport  InitialOutput=0
  wires:
  In Q/1 -> IS-95A Rev Ch  Rake Finger2/2, IS-95A Rev Ch  Rake Finger3/2, IS-95A Rev Ch  Rake Finger1/2
  In I/1 -> IS-95A Rev Ch  Rake Finger2/1, IS-95A Rev Ch  Rake Finger3/1, IS-95A Rev Ch  Rake Finger1/1
  IS-95A Rev Ch  Rake Finger2/1 -> Rake Combiner/2
  [P1] -> Demux1/1
  Demux1/1 -> IS-95A Rev Ch  Rake Finger1/6
  Demux1/2 -> IS-95A Rev Ch  Rake Finger1/Enable
  [P2] -> Demux2/1
  Demux2/1 -> IS-95A Rev Ch  Rake Finger2/6
  Demux2/2 -> IS-95A Rev Ch  Rake Finger2/Enable
  [P3] -> Demux3/1
  Demux3/1 -> IS-95A Rev Ch  Rake Finger3/6
  Demux3/2 -> IS-95A Rev Ch  Rake Finger3/Enable
  Unipolar to Bipolar Converter/1 -> Integer Delay/1
  LC/1 -> Unipolar to Bipolar Converter/1
  Integer Delay/1 -> IS-95A Rev Ch  Rake Finger2/5, IS-95A Rev Ch  Rake Finger3/5, IS-95A Rev Ch  Rake Finger1/5
  Integer Delay2/1 -> IS-95A Rev Ch  Rake Finger1/3, IS-95A Rev Ch  Rake Finger2/3, IS-95A Rev Ch  Rake Finger3/3
  Sync Delay/1 -> IS-95A Rev Ch  Rake Finger1/4, IS-95A Rev Ch  Rake Finger2/4, IS-95A Rev Ch  Rake Finger3/4
  Short PN Mask/1 -> IS-95A Short Code Generator/1
  IS-95A Short Code Generator/2 -> Sync Delay/1
  IS-95A Short Code Generator/1 -> Integer Delay2/1
  Initial Phases/Enables/1 -> Demux/1
  Demux/1 -> [P1]
  Demux/2 -> [P2]
  Demux/3 -> [P3]
  IS-95A Rev Ch  Rake Finger3/1 -> Rake Combiner/3
  IS-95A Rev Ch  Rake Finger1/1 -> Rake Combiner/1
  Rake Combiner/1 -> Gain/1
  Gain/1 -> Rake Out/1

== system cdmalibv1p1/IS-95A Base Station Receiver/IS-95A Rev Ch Detector/Rev Ch Randomizer Gating Signal Generator ==
  Rate : Inport
  LC : Inport  Port=2
  Buffer1 : dspbuff3/Buffer  N=16  V=0  ic=0
  Buffer2 : dspbuff3/Buffer  N=1536  V=0  ic=0
  Down-Sampler : Selector  InputPortWidth=1536
  IS-95A Rev Ch Burst Randomizer : cdmalibv1p1/IS-95A Mobile Station Transmitter/IS-95A Rev Ch Burst Randomizer  chType=Traffic  initLCSt=[]
  Sync Delay : dspsigops/Integer Delay  delay=15  ic=0
  Gating Sig : Outport  InitialOutput=0
  wires:
  Buffer1/1 -> Gating Sig/1
  IS-95A Rev Ch Burst Randomizer/1 -> Buffer2/1
  Down-Sampler/1 -> Sync Delay/1
  Buffer2/1 -> Down-Sampler/1
  Sync Delay/1 -> Buffer1/1
  LC/1 -> IS-95A Rev Ch Burst Randomizer/2
  Rate/1 -> IS-95A Rev Ch Burst Randomizer/1

== system cdmalibv1p1/IS-95A Base Station Receiver/IS-95A Rev Ch Detector/Rev Ch Walsh Demodulator ==
  Data In : Inport
  Buffer : dspbuff3/Buffer  N=576  V=0  ic=0
  Buffer1 : dspbuff3/Buffer  N=576  V=0  ic=0
  IS-95A Rev Ch Walsh Demodulator : cdmalibv1p1/IS-95A Base Station Receiver/IS-95A Rev Ch Walsh Demodulator  wlshOrd=wlshOrder  numSymb=1
  Integer Delay2 : dspsigops/Integer Delay  delay=((576 - off * wlshOrder)* wlshOrder) / (inSize * wlshOrder)  ic=0
  Integer Delay3 : dspsigops/Integer Delay  delay=((576 - off * wlshOrder)* wlshOrder) / (inSize * wlshOrder)  ic=0
  Hard Decision : Outport  InitialOutput=0
  Soft Decision : Outport  Port=2  InitialOutput=0
  wires:
  Buffer/1 -> Hard Decision/1
  Data In/1 -> IS-95A Rev Ch Walsh Demodulator/1
  IS-95A Rev Ch Walsh Demodulator/1 -> Integer Delay2/1
  Integer Delay2/1 -> Buffer/1
  IS-95A Rev Ch Walsh Demodulator/2 -> Integer Delay3/1
  Integer Delay3/1 -> Buffer1/1
  Buffer1/1 -> Soft Decision/1

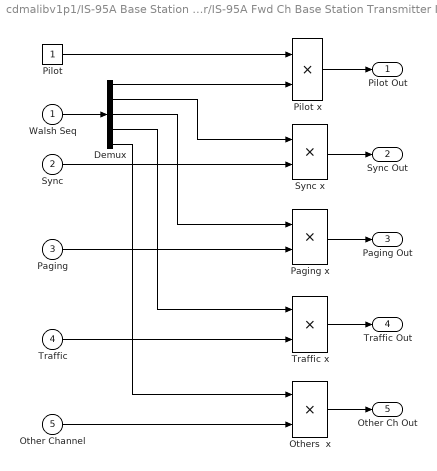
== system cdmalibv1p1/IS-95A Base Station Transmitter/IS-95A Fwd Ch Base Station Transmitter Interface/Walsh Mixer ==
  Walsh Seq : Inport
  Sync : Inport  Port=2
  Paging : Inport  Port=3
  Traffic : Inport  Port=4  SampleTime=1/50/384
  Other Channel : Inport  Port=5
  "Demux " : Demux  Outputs=[64 64 64 64 -1]
  Others  x : Product  Inputs=**  SaturateOnIntegerOverflow=on  InputSameDT=on
  Paging x : Product  Inputs=**  SaturateOnIntegerOverflow=on  InputSameDT=on
  Pilot : Constant
  Pilot x : Product  Inputs=**  SaturateOnIntegerOverflow=on  InputSameDT=on
  Sync x : Product  Inputs=**  SaturateOnIntegerOverflow=on  InputSameDT=on
  Traffic x : Product  Inputs=**  SaturateOnIntegerOverflow=on  InputSameDT=on
  Pilot Out : Outport  InitialOutput=0
  Sync Out : Outport  Port=2  InitialOutput=0
  Paging Out : Outport  Port=3  InitialOutput=0
  Traffic Out : Outport  Port=4  InitialOutput=0
  Other Ch Out : Outport  Port=5  InitialOutput=0
  wires:
  Walsh Seq/1 -> "Demux "/1
  Other Channel/1 -> Others  x/2
  "Demux "/1 -> Pilot x/2
  Sync/1 -> Sync x/2
  Pilot/1 -> Pilot x/1
  "Demux "/2 -> Sync x/1
  Traffic/1 -> Traffic x/2
  Paging/1 -> Paging x/2
  "Demux "/5 -> Others  x/1
  "Demux "/4 -> Traffic x/1
  "Demux "/3 -> Paging x/1
  Others  x/1 -> Other Ch Out/1
  Sync x/1 -> Sync Out/1
  Pilot x/1 -> Pilot Out/1
  Traffic x/1 -> Traffic Out/1
  Paging x/1 -> Paging Out/1

== system cdmalibv1p1/IS-95A Common/IS-95A Frame Quality  Detector/Sync Channel Detection  Logic and Offset Correction ==
  Rate : Inport
  Channel Type : Constant  Value=chType-1
  Logical Operator : Logic  Operator=NOT
  Logical Operator1 : Logic
  Product : Product  SaturateOnIntegerOverflow=on  InputSameDT=on
  Relational Operator : RelationalOperator  Operator===
  Sync Channel  Offset : Constant  Value=3
  "Sync or Traffic Eigth rate " : Constant  Value=3
  Sync Offset : Outport  InitialOutput=0
  wires:
  Product/1 -> Sync Offset/1
  Sync Channel  Offset/1 -> Product/1
  Logical Operator1/1 -> Product/2
  Relational Operator/1 -> Logical Operator1/2
  "Sync or Traffic Eigth rate "/1 -> Relational Operator/2
  Rate/1 -> Relational Operator/1
  Logical Operator/1 -> Logical Operator1/1
  Channel Type/1 -> Logical Operator/1

== system cdmalibv1p1/IS-95A Mobile Station Receiver/IS-95A Fwd Ch Descrambler/Start Time FR ==
  Digital Clock : DigitalClock  SampleTime=1/50/384
  Relational Operator : RelationalOperator
  Start time : Constant  Value=rake_buff_size*(1/50/384)
  Enable : Outport  InitialOutput=0
  wires:
  Relational Operator/1 -> Enable/1
  Start time/1 -> Relational Operator/2
  Digital Clock/1 -> Relational Operator/1

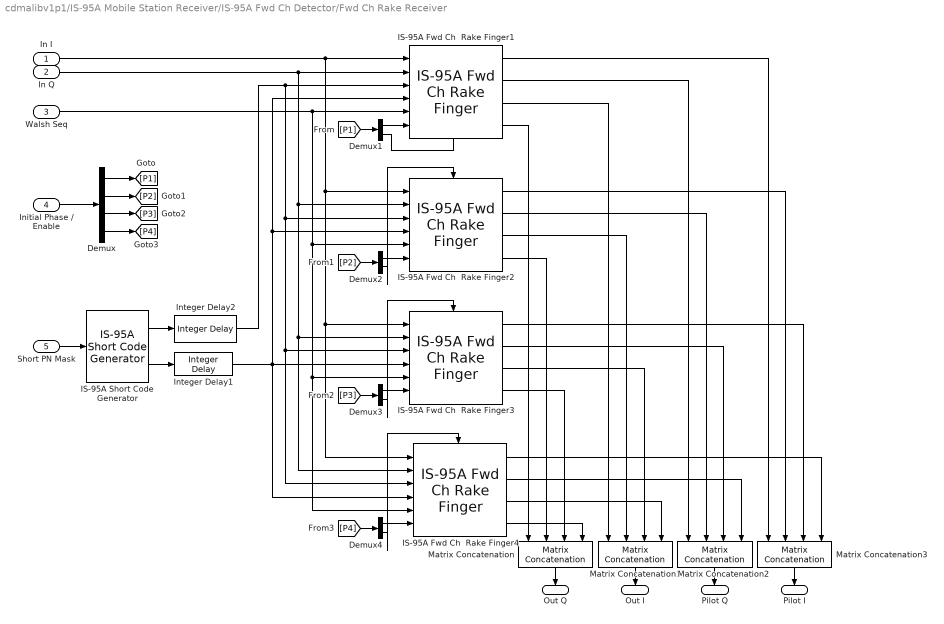
== system cdmalibv1p1/IS-95A Mobile Station Receiver/IS-95A Fwd Ch Detector/Fwd Ch Rake Receiver  ==
  In I : Inport
  In Q : Inport  Port=2
  Walsh Seq : Inport  Port=3
  Initial Phase / Enable : Inport  Port=4
  Short PN Mask : Inport  Port=5
  Demux : Demux
  Demux{1..4} (4 alike) : Demux  Outputs=2
  IS-95A Fwd Ch  Rake Finger{1..4} (4 alike) : cdmalibv1p1/IS-95A Mobile Station Receiver/IS-95A Fwd Ch  Rake Finger  wlshOrd=wlshOrd  numSymb=numSymb  buffSize=rake_buff_size  ovrSmp=rake_oversamp
  IS-95A Short Code Generator : cdmalibv1p1/IS-95A Common/IS-95A Short Code Generator  numOut=64  sampTime=1/(50*384)
  Integer Delay1 : dspsigops/Integer Delay  delay=rake_buff_size*(2^wlshOrd)  ic=0
  Integer Delay2 : dspsigops/Integer Delay  delay=rake_buff_size*(2^wlshOrd)  ic=0
  Matrix Concatenation{,1..3} (4 alike) : simulink3/Signals & Systems/Matrix Concatenation  Orientation=down  numInports=4  catMethod=Vertical
  Pilot I : Outport  Orientation=down  InitialOutput=0
  Pilot Q : Outport  Orientation=down  Port=2  InitialOutput=0
  Out I : Outport  Orientation=down  Port=3  InitialOutput=0
  Out Q : Outport  Orientation=down  Port=4  InitialOutput=0
  wires:
  Matrix Concatenation3/1 -> Pilot I/1
  Matrix Concatenation2/1 -> Pilot Q/1
  Matrix Concatenation1/1 -> Out I/1
  Matrix Concatenation/1 -> Out Q/1
  Short PN Mask/1 -> IS-95A Short Code Generator/1
  IS-95A Fwd Ch  Rake Finger4/4 -> Matrix Concatenation/4
  IS-95A Fwd Ch  Rake Finger3/4 -> Matrix Concatenation/3
  IS-95A Fwd Ch  Rake Finger2/4 -> Matrix Concatenation/2
  IS-95A Fwd Ch  Rake Finger1/4 -> Matrix Concatenation/1
  IS-95A Fwd Ch  Rake Finger1/3 -> Matrix Concatenation1/1
  IS-95A Fwd Ch  Rake Finger3/3 -> Matrix Concatenation1/3
  IS-95A Fwd Ch  Rake Finger4/3 -> Matrix Concatenation1/4
  IS-95A Fwd Ch  Rake Finger4/2 -> Matrix Concatenation2/4
  IS-95A Fwd Ch  Rake Finger3/2 -> Matrix Concatenation2/3
  IS-95A Fwd Ch  Rake Finger2/2 -> Matrix Concatenation2/2
  IS-95A Fwd Ch  Rake Finger1/2 -> Matrix Concatenation2/1
  IS-95A Fwd Ch  Rake Finger1/1 -> Matrix Concatenation3/1
  IS-95A Fwd Ch  Rake Finger2/1 -> Matrix Concatenation3/2
  IS-95A Fwd Ch  Rake Finger3/1 -> Matrix Concatenation3/3
  IS-95A Fwd Ch  Rake Finger4/1 -> Matrix Concatenation3/4
  Demux2/2 -> IS-95A Fwd Ch  Rake Finger2/Enable
  Demux2/1 -> IS-95A Fwd Ch  Rake Finger2/6
  Demux3/2 -> IS-95A Fwd Ch  Rake Finger3/Enable
  Demux3/1 -> IS-95A Fwd Ch  Rake Finger3/6
  Walsh Seq/1 -> IS-95A Fwd Ch  Rake Finger1/5, IS-95A Fwd Ch  Rake Finger2/5, IS-95A Fwd Ch  Rake Finger4/5, IS-95A Fwd Ch  Rake Finger3/5
  Demux4/1 -> IS-95A Fwd Ch  Rake Finger4/6
  Demux1/2 -> IS-95A Fwd Ch  Rake Finger1/Enable
  Demux1/1 -> IS-95A Fwd Ch  Rake Finger1/6
  [P1] -> Demux1/1
  Integer Delay1/1 -> IS-95A Fwd Ch  Rake Finger1/4, IS-95A Fwd Ch  Rake Finger2/4, IS-95A Fwd Ch  Rake Finger3/4, IS-95A Fwd Ch  Rake Finger4/4
  In I/1 -> IS-95A Fwd Ch  Rake Finger1/1, IS-95A Fwd Ch  Rake Finger2/1, IS-95A Fwd Ch  Rake Finger3/1, IS-95A Fwd Ch  Rake Finger4/1
  In Q/1 -> IS-95A Fwd Ch  Rake Finger1/2, IS-95A Fwd Ch  Rake Finger2/2, IS-95A Fwd Ch  Rake Finger3/2, IS-95A Fwd Ch  Rake Finger4/2
  IS-95A Fwd Ch  Rake Finger2/3 -> Matrix Concatenation1/2
  Demux4/2 -> IS-95A Fwd Ch  Rake Finger4/Enable
  [P4] -> Demux4/1
  [P3] -> Demux3/1
  [P2] -> Demux2/1
  Integer Delay2/1 -> IS-95A Fwd Ch  Rake Finger1/3, IS-95A Fwd Ch  Rake Finger2/3, IS-95A Fwd Ch  Rake Finger3/3, IS-95A Fwd Ch  Rake Finger4/3
  IS-95A Short Code Generator/2 -> Integer Delay1/1
  IS-95A Short Code Generator/1 -> Integer Delay2/1
  Demux/4 -> [P4]
  Demux/3 -> [P3]
  Demux/2 -> [P2]
  Demux/1 -> [P1]
  Initial Phase / Enable/1 -> Demux/1
